simulink model "BC_K9"  (R2025a)
settings: Solver=VariableStepAuto  StartTime=0.0  StopTime=2  MaxStep=1e-3  RelTol=1e-3
libraries: simulink_extras x1
settings Model: Creator=Szalay  LastModifiedBy=Szalay

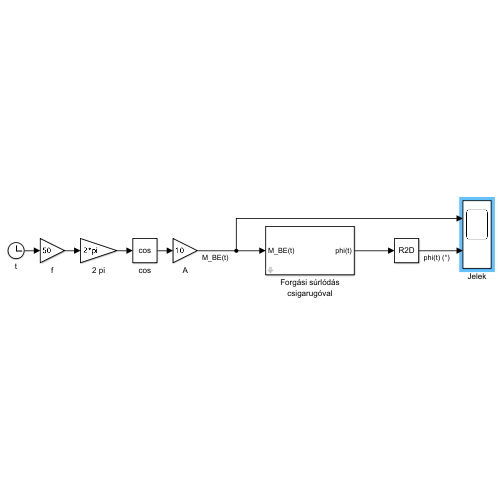
[thumbnail: Simulink's stored preview of the top-level diagram]
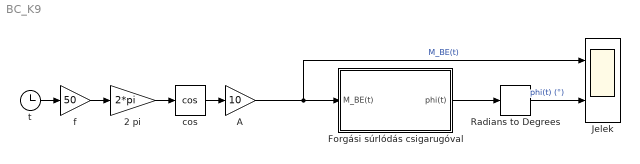
== system BC_K9 ==
  2 pi : Gain  Gain=2*pi
  A : Gain  Gain=10
  Forgási súrlódás csigarugóval : Subsystem  mask(Forgási súrlódás csigarugóval){B=0.1, C=0.5, phi_0=30}
      mask prompts: B "Forgási súrlódási együttható (Nms/rad)"; C "Csavarási rugómerevség (Nm/rad)"; phi_0 "Kezdeti szöghelyzet (°)"
      mask help: Csigarugó ellenében forgó, surlódó, elhanyagolható tehetetlenségi nyomatékú tengely forgómozgásának modellje.
      mask DialogControl ParameterGroupVar Prompt: Modellparaméterek
      mask DialogControl Container3 Prompt: Kezdeti érték
  Jelek : Scope  NumInputPorts=2
      settings: ActiveDisplayYMinimum=-26.411971296436185  ActiveDisplayYMaximum=55.389626229730453
  Radians to Degrees : simulink_extras/Transformations/Radians to Degrees
  cos : Trigonometry  Operator=cos
  f : Gain  Gain=50
  t : Clock
  wires:
  t/1 -> f/1
  f/1 -> 2 pi/1
  2 pi/1 -> cos/1
  cos/1 -> A/1
  A/1 -> Jelek/1, Forgási súrlódás csigarugóval/1(M_BE(t))  "M_BE(t)"
  Forgási súrlódás csigarugóval/1(phi(t)) -> Radians to Degrees/1
  Radians to Degrees/1 -> Jelek/2  "phi(t) (°)"

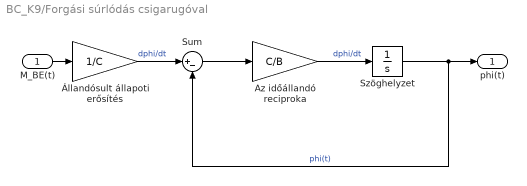
== system BC_K9/Forgási súrlódás csigarugóval ==
  M_BE(t) : Inport
  Az időállandó reciproka : Gain  Gain=C/B
  Sum : Sum  Inputs=|+-
  Szöghelyzet : Integrator  InitialCondition=phi_0 * pi/180
  Állandósult állapoti erősítés : Gain  Gain=1/C
  phi(t) : Outport
  wires:
  Szöghelyzet/1 -> phi(t)/1, Sum/2  "phi(t)"
  M_BE(t)/1 -> Állandósult állapoti erősítés/1
  Állandósult állapoti erősítés/1 -> Sum/1  "dphi/dt"
  Sum/1 -> Az időállandó reciproka/1
  Az időállandó reciproka/1 -> Szöghelyzet/1  "dphi/dt"
